simulink model "nonlinearities"  (R2018a)
settings: Solver=VariableStepAuto  StartTime=0.0  StopTime=20  RelTol=1e-3
libraries: simulink x6
settings Model: Creator=maria  LastModifiedBy=maria

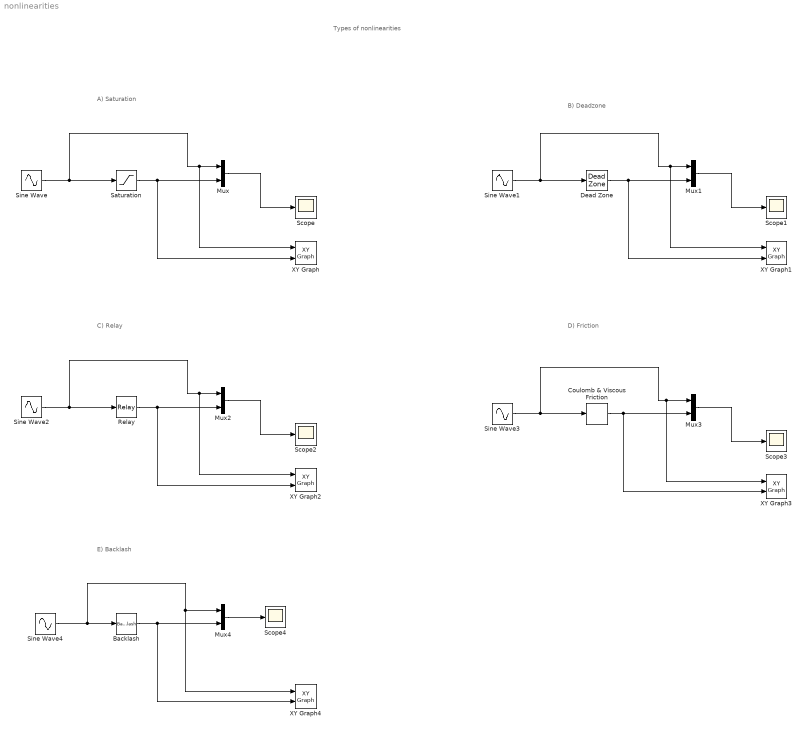
== system nonlinearities ==
  note: A) Saturation
  note: Types of nonlinearities
  note: B) Deadzone
  note: C) Relay
  note: D) Friction
  note: E) Backlash
  Backlash : Backlash
  Coulomb & Viscous Friction : simulink/Discontinuities/Coulomb & Viscous Friction  offset=[1]  gain=1
      settings: SourceProductName=Simulink
  Dead Zone : DeadZone  SaturateOnIntegerOverflow=on
  Mux{,1..4} (5 alike) : Mux  Inputs=2
  Relay : Relay
  Saturation : Saturate
  Scope{,1..4} (5 alike) : Scope
  Sine Wave{,1..4} (5 alike) : Sin  SampleTime=0
  XY Graph : simulink/Sinks/XY Graph  xmin=-1  xmax=1  ymin=-1  ymax=1  st=-1
  XY Graph1 : simulink/Sinks/XY Graph  xmin=-1  xmax=1  ymin=-1  ymax=1  st=-1
  XY Graph2 : simulink/Sinks/XY Graph  xmin=-1  xmax=1  ymin=-1.5  ymax=1.5  st=-1
  XY Graph3 : simulink/Sinks/XY Graph  xmin=-1  xmax=1  ymin=-2  ymax=2  st=-1
  XY Graph4 : simulink/Sinks/XY Graph  xmin=-2  xmax=2  ymin=-2  ymax=2  st=-1
  wires:
  Sine Wave/1 -> XY Graph/1, Mux/1, Saturation/1
  Saturation/1 -> XY Graph/2, Mux/2
  Mux/1 -> Scope/1
  Mux1/1 -> Scope1/1
  Dead Zone/1 -> Mux1/2, XY Graph1/2
  Sine Wave1/1 -> Dead Zone/1, Mux1/1, XY Graph1/1
  Sine Wave2/1 -> Relay/1, XY Graph2/1, Mux2/1
  Relay/1 -> XY Graph2/2, Mux2/2
  Mux2/1 -> Scope2/1
  Mux3/1 -> Scope3/1
  Coulomb & Viscous Friction/1 -> XY Graph3/2, Mux3/2
  Sine Wave3/1 -> Coulomb & Viscous Friction/1, XY Graph3/1, Mux3/1
  Backlash/1 -> XY Graph4/2, Mux4/2
  Mux4/1 -> Scope4/1
  Sine Wave4/1 -> XY Graph4/1, Mux4/1, Backlash/1
